simulink model "ALL_SET_GET_SETUP_Funcitons_Library_2020a"  (R2021b)
settings: Solver=VariableStepAuto  StartTime=0.0  StopTime=inf  RelTol=1e-3
(part 1 of 3)
settings Model: Creator=ccortez  LastModifiedBy=SL_1
settings SolverCC: AlgebraicLoopSolver=TrustRegion
settings DebuggingCC: SFMachineParentedDataDiag=warning

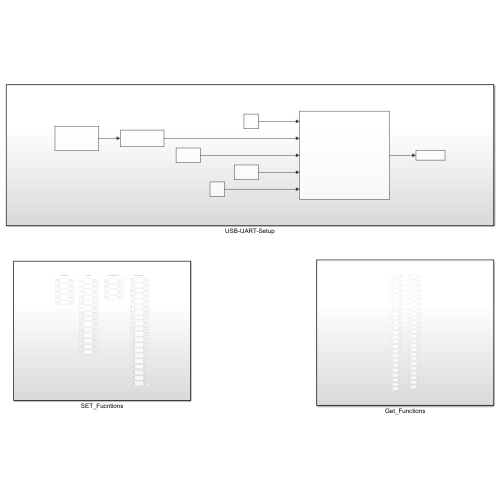
[thumbnail: Simulink's stored preview of the top-level diagram]
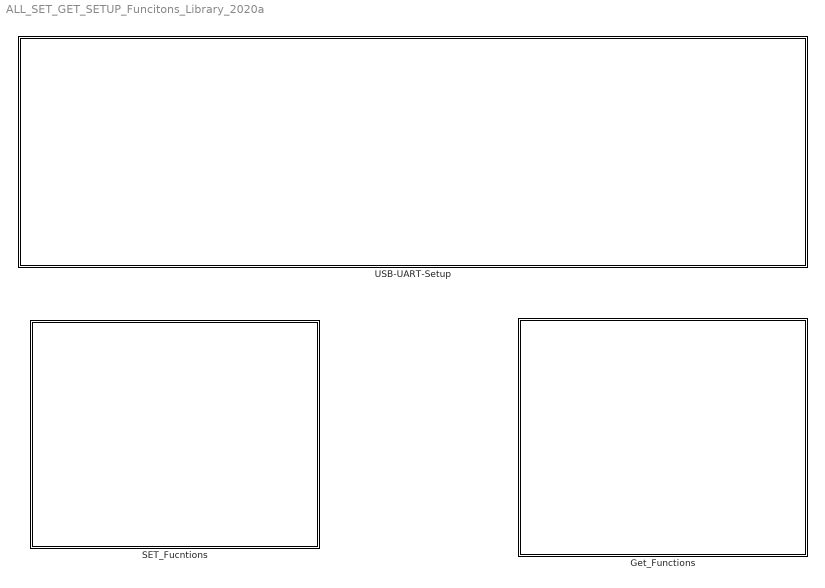
== system ALL_SET_GET_SETUP_Funcitons_Library_2020a ==
  Get_Functions : Subsystem
  SET_Fucntions : Subsystem
  USB-UART-Setup : Subsystem

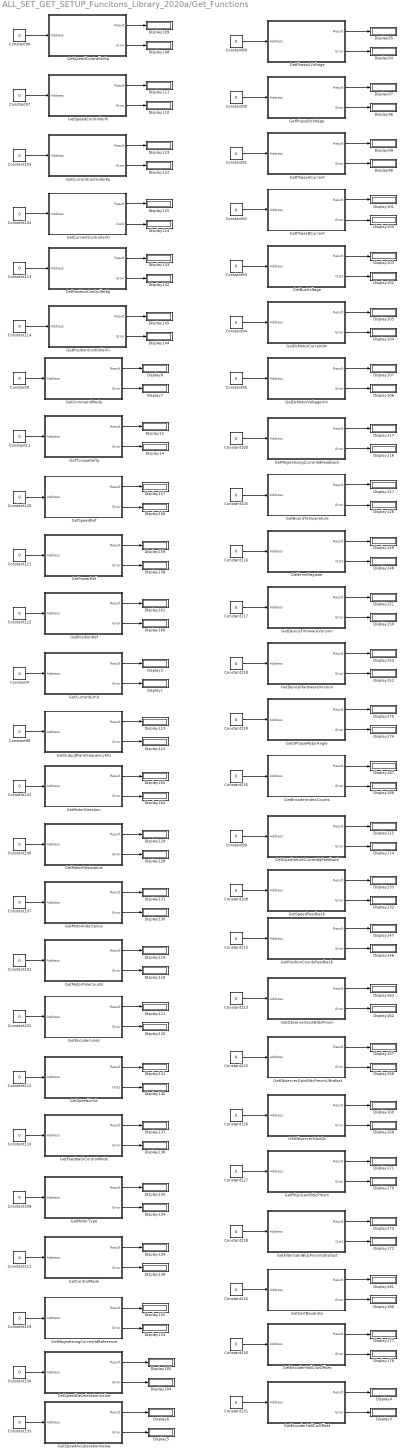
== system ALL_SET_GET_SETUP_Funcitons_Library_2020a/Get_Functions ==
  Constant{4,8,11,89..135} (50 alike) : Constant  Value=0  OutDataTypeStr=uint8
  Display{1..8,14..15,94..177,180..181,184..187} (100 alike) : Display
      settings: Format=decimal (Stored Integer)
  Get3PhaseMotorAngle : Subsystem
  GetBoardTemperature : Subsystem
  GetBusVoltage : Subsystem
  GetCommandMode : Subsystem
  GetControlMode : Subsystem
  GetCurrentControllerKi : Subsystem
  GetCurrentControllerKp : Subsystem
  GetCurrentLimit : Subsystem
  GetDcMotorCurrentIm : Subsystem
  GetDcMotorVoltageVm : Subsystem
  GetDeviceFirmwareVersion : Subsystem
  GetDeviceHardwareVersion : Subsystem
  GetEncoderHallCcwOffset : Subsystem
  GetEncoderHallCwOffset : Subsystem
  GetEncoderIndexCounts : Subsystem
  GetEncoderLines : Subsystem
  GetErrorRegister : Subsystem
  GetFeedbackControlMode : Subsystem
  GetFilterGainBldcPmsm : Subsystem
  GetFilterGainBldcPmsmUltrafast : Subsystem
  GetMagnetizingCurrentIdFeedback : Subsystem
  GetMagnetizingCurrentIdReference : Subsystem
  GetMotorDirection : Subsystem
  GetMotorInductance : Subsystem
  GetMotorPoleCounts : Subsystem
  GetMotorResistance : Subsystem
  GetMotorType : Subsystem
  GetObserverGainBldcPmsm : Subsystem
  GetObserverGainBldcPmsmUltrafast : Subsystem
  GetObserverGainDc : Subsystem
  GetOutputPwmFrequencyKhz : Subsystem
  GetPhaseACurrent : Subsystem
  GetPhaseAVoltage : Subsystem
  GetPhaseBCurrent : Subsystem
  GetPhaseBVoltage : Subsystem
  GetPositionControllerKi : Subsystem
  GetPositionControllerKp : Subsystem
  GetPositionCountsFeedback : Subsystem
  GetPositionRef : Subsystem
  GetPowerRef : Subsystem
  GetQuadratureCurrentIqFeedback : Subsystem
  GetSpeedAccelerationValue : Subsystem
  GetSpeedControllerKi : Subsystem
  GetSpeedControllerKp : Subsystem
  GetSpeedDecelerationValue : Subsystem
  GetSpeedFeedback : Subsystem
  GetSpeedLimit : Subsystem
  GetSpeedRef : Subsystem
  GetTorqueRefIq : Subsystem
  GetUartBaudrate : Subsystem
  wires:
  GetErrorRegister/1(Result) -> Display149/1
  Get3PhaseMotorAngle/2(Error) -> Display174/1
  GetDeviceHardwareVersion/1(Result) -> Display153/1
  Constant91/1 -> GetPhaseACurrent/1(Address)
  GetMagnetizingCurrentIdFeedback/2(Error) -> Display116/1
  Constant129/1 -> Get3PhaseMotorAngle/1(Address)
  GetDcMotorVoltageVm/2(Error) -> Display106/1
  GetPhaseACurrent/1(Result) -> Display99/1
  GetBusVoltage/1(Result) -> Display103/1
  GetErrorRegister/2(Out2) -> Display148/1
  Get3PhaseMotorAngle/1(Result) -> Display175/1
  Constant99/1 -> GetQuadratureCurrentIqFeedback/1(Address)
  Constant117/1 -> GetDeviceFirmwareVersion/1(Address)
  GetPhaseAVoltage/2(Error) -> Display94/1
  Constant116/1 -> GetErrorRegister/1(Address)
  GetPhaseACurrent/2(Error) -> Display98/1
  GetBoardTemperature/1(Result) -> Display127/1
  GetBusVoltage/2(Out2) -> Display102/1
  GetMagnetizingCurrentIdFeedback/1(Result) -> Display117/1
  GetBoardTemperature/2(Error) -> Display126/1
  Constant100/1 -> GetMagnetizingCurrentIdFeedback/1(Address)
  GetPositionCountsFeedback/2(Error) -> Display146/1
  GetPositionCountsFeedback/1(Result) -> Display147/1
  Constant105/1 -> GetBoardTemperature/1(Address)
  GetPhaseBVoltage/1(Result) -> Display97/1
  Constant90/1 -> GetPhaseBVoltage/1(Address)
  GetPhaseBVoltage/2(Error) -> Display96/1
  GetQuadratureCurrentIqFeedback/1(Result) -> Display115/1
  GetDeviceFirmwareVersion/1(Result) -> Display151/1
  GetDcMotorVoltageVm/1(Result) -> Display107/1
  Constant92/1 -> GetPhaseBCurrent/1(Address)
  GetEncoderIndexCounts/1(Result) -> Display187/1
  GetSpeedFeedback/2(Error) -> Display132/1
  GetQuadratureCurrentIqFeedback/2(Error) -> Display114/1
  Constant89/1 -> GetPhaseAVoltage/1(Address)
  GetDeviceFirmwareVersion/2(Error) -> Display150/1
  GetPhaseBCurrent/1(Result) -> Display101/1
  Constant95/1 -> GetDcMotorVoltageVm/1(Address)
  GetPhaseBCurrent/2(Error) -> Display100/1
  GetPhaseAVoltage/1(Result) -> Display95/1
  Constant118/1 -> GetDeviceHardwareVersion/1(Address)
  Constant108/1 -> GetSpeedFeedback/1(Address)
  GetSpeedFeedback/1(Result) -> Display133/1
  GetDcMotorCurrentIm/2(Error) -> Display104/1
  Constant93/1 -> GetBusVoltage/1(Address)
  GetEncoderIndexCounts/2(Error) -> Display186/1
  Constant115/1 -> GetPositionCountsFeedback/1(Address)
  GetDcMotorCurrentIm/1(Result) -> Display105/1
  Constant94/1 -> GetDcMotorCurrentIm/1(Address)
  GetDeviceHardwareVersion/2(Error) -> Display152/1
  Constant135/1 -> GetEncoderIndexCounts/1(Address)
  GetObserverGainBldcPmsmUltrafast/2(Error) -> Display166/1
  GetObserverGainBldcPmsmUltrafast/1(Result) -> Display167/1
  Constant125/1 -> GetObserverGainBldcPmsmUltrafast/1(Address)
  GetPositionControllerKi/1(Result) -> Display145/1
  GetPositionControllerKi/2(Error) -> Display144/1
  GetEncoderHallCcwOffset/1(Result) -> Display177/1
  GetEncoderHallCcwOffset/2(Error) -> Display176/1
  GetUartBaudrate/1(Result) -> Display181/1
  Constant132/1 -> GetUartBaudrate/1(Address)
  Constant126/1 -> GetObserverGainDc/1(Address)
  GetControlMode/1(Result) -> Display139/1
  GetControlMode/2(Error) -> Display138/1
  Constant111/1 -> GetControlMode/1(Address)
  GetFeedbackControlMode/2(Error) -> Display136/1
  GetFeedbackControlMode/1(Result) -> Display137/1
  GetSpeedAccelerationValue/2(Error) -> Display5/1
  GetObserverGainDc/1(Result) -> Display169/1
  GetObserverGainBldcPmsm/2(Error) -> Display162/1
  Constant123/1 -> GetObserverGainBldcPmsm/1(Address)
  GetObserverGainBldcPmsm/1(Result) -> Display163/1
  Constant110/1 -> GetFeedbackControlMode/1(Address)
  GetMotorDirection/2(Error) -> Display164/1
  GetEncoderLines/2(Error) -> Display120/1
  Constant119/1 -> GetMagnetizingCurrentIdReference/1(Address)
  Constant122/1 -> GetPositionRef/1(Address)
  Constant107/1 -> GetMotorInductance/1(Address)
  GetMotorInductance/1(Result) -> Display131/1
  Constant127/1 -> GetFilterGainBldcPmsm/1(Address)
  GetSpeedLimit/2(Out2) -> Display140/1
  Constant112/1 -> GetSpeedLimit/1(Address)
  GetFilterGainBldcPmsmUltrafast/2(Out2) -> Display172/1
  GetMotorInductance/2(Error) -> Display130/1
  GetUartBaudrate/2(Error) -> Display180/1
  Constant133/1 -> GetSpeedAccelerationValue/1(Address)
  Constant128/1 -> GetFilterGainBldcPmsmUltrafast/1(Address)
  GetPositionRef/1(Result) -> Display161/1
  Constant124/1 -> GetMotorDirection/1(Address)
  GetMagnetizingCurrentIdReference/2(Error) -> Display154/1
  Constant130/1 -> GetEncoderHallCcwOffset/1(Address)
  GetFilterGainBldcPmsmUltrafast/1(Result) -> Display173/1
  Constant131/1 -> GetEncoderHallCwOffset/1(Address)
  Constant102/1 -> GetEncoderLines/1(Address)
  GetCurrentControllerKp/2(Error) -> Display122/1
  Constant113/1 -> GetPositionControllerKp/1(Address)
  GetCurrentControllerKp/1(Result) -> Display123/1
  Constant98/1 -> GetOutputPwmFrequencyKhz/1(Address)
  GetSpeedDecelerationValue/2(Error) -> Display184/1
  GetObserverGainDc/2(Error) -> Display168/1
  Constant114/1 -> GetPositionControllerKi/1(Address)
  GetSpeedAccelerationValue/1(Result) -> Display6/1
  GetFilterGainBldcPmsm/2(Error) -> Display170/1
  GetPositionRef/2(Error) -> Display160/1
  Constant134/1 -> GetSpeedDecelerationValue/1(Address)
  GetOutputPwmFrequencyKhz/2(Error) -> Display112/1
  Constant104/1 -> GetCurrentControllerKi/1(Address)
  GetCurrentControllerKi/2(Out2) -> Display124/1
  GetCurrentControllerKi/1(Result) -> Display125/1
  Constant103/1 -> GetCurrentControllerKp/1(Address)
  GetPositionControllerKp/1(Result) -> Display143/1
  GetMotorPoleCounts/2(Error) -> Display118/1
  GetPositionControllerKp/2(Error) -> Display142/1
  GetSpeedDecelerationValue/1(Result) -> Display185/1
  GetFilterGainBldcPmsm/1(Result) -> Display171/1
  GetOutputPwmFrequencyKhz/1(Result) -> Display113/1
  GetEncoderLines/1(Result) -> Display121/1
  GetMotorPoleCounts/1(Result) -> Display119/1
  GetMotorResistance/1(Result) -> Display129/1
  Constant101/1 -> GetMotorPoleCounts/1(Address)
  GetMotorDirection/1(Result) -> Display165/1
  GetMagnetizingCurrentIdReference/1(Result) -> Display155/1
  GetMotorType/1(Result) -> Display135/1
  GetMotorType/2(Error) -> Display134/1
  GetSpeedLimit/1(Result) -> Display141/1
  Constant109/1 -> GetMotorType/1(Address)
  Constant106/1 -> GetMotorResistance/1(Address)
  GetMotorResistance/2(Error) -> Display128/1
  GetPowerRef/2(Error) -> Display158/1
  Constant121/1 -> GetPowerRef/1(Address)
  Constant120/1 -> GetSpeedRef/1(Address)
  GetSpeedRef/1(Result) -> Display157/1
  GetSpeedRef/2(Error) -> Display156/1
  GetTorqueRefIq/1(Result) -> Display15/1
  Constant8/1 -> GetCommandMode/1(Address)
  GetCommandMode/2(Error) -> Display7/1
  GetTorqueRefIq/2(Error) -> Display14/1
  GetPowerRef/1(Result) -> Display159/1
  Constant11/1 -> GetTorqueRefIq/1(Address)
  GetCommandMode/1(Result) -> Display8/1
  Constant4/1 -> GetCurrentLimit/1(Address)
  GetCurrentLimit/1(Result) -> Display2/1
  GetCurrentLimit/2(Error) -> Display1/1
  GetSpeedControllerKi/1(Result) -> Display111/1
  GetSpeedControllerKp/2(Error) -> Display108/1
  GetSpeedControllerKp/1(Result) -> Display109/1
  GetSpeedControllerKi/2(Error) -> Display110/1
  Constant97/1 -> GetSpeedControllerKi/1(Address)
  Constant96/1 -> GetSpeedControllerKp/1(Address)
  GetEncoderHallCwOffset/2(Error) -> Display3/1
  GetEncoderHallCwOffset/1(Result) -> Display4/1

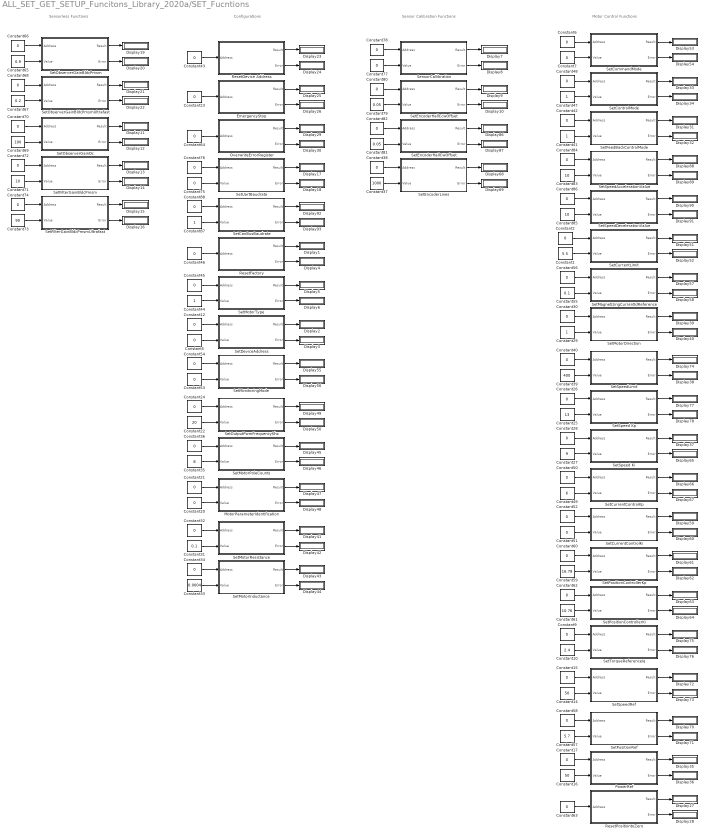
== system ALL_SET_GET_SETUP_Funcitons_Library_2020a/SET_Fucntions ==
  note: Sensor Calibration Functions
  note: Sensorless Functions
  note: Configurations
  note: Motor Control Functions
  Constant1 : Constant  Value=5.5  OutDataTypeStr=single
  Constant10 : Constant  Value=2.4  OutDataTypeStr=single
  Constant{2,5..6,9,12,15,17,21,23..24,26,28,30,32,34,36,38,40,42..43,45..46,48,50,52,54,56,58,60,62..64,66,68,70,72,74,76..78,80,82,84,86,88} (45 alike) : Constant  Value=0  OutDataTypeStr=uint8
  Constant14 : Constant  Value=50  OutDataTypeStr=uint32
  Constant16 : Constant  Value=50  OutDataTypeStr=single
  Constant{7,20,53,75} (4 alike) : Constant  Value=0  OutDataTypeStr=boolean
  Constant22 : Constant  Value=20  OutDataTypeStr=uint32
  Constant25 : Constant  Value=13  OutDataTypeStr=single
  Constant27 : Constant  Value=9  OutDataTypeStr=single
  Constant29 : Constant  OutDataTypeStr=boolean
  Constant31 : Constant  Value=0.1  OutDataTypeStr=single
  Constant33 : Constant  Value=0.0004  OutDataTypeStr=single
  Constant35 : Constant  Value=8  OutDataTypeStr=uint32
  Constant37 : Constant  Value=1000  OutDataTypeStr=uint32
  Constant39 : Constant  Value=400  OutDataTypeStr=uint32
  Constant{41,44,47,87} (4 alike) : Constant  OutDataTypeStr=uint8
  Constant49 : Constant  Value=6  OutDataTypeStr=single
  Constant51 : Constant  Value=0  OutDataTypeStr=single
  Constant55 : Constant  Value=0.1  OutDataTypeStr=single
  Constant57 : Constant  Value=5.7  OutDataTypeStr=uint32
  Constant59 : Constant  Value=16.78  OutDataTypeStr=single
  Constant61 : Constant  Value=10.76  OutDataTypeStr=single
  Constant65 : Constant  Value=0.9  OutDataTypeStr=single
  Constant67 : Constant  Value=0.2  OutDataTypeStr=single
  Constant69 : Constant  Value=100  OutDataTypeStr=single
  Constant71 : Constant  Value=10  OutDataTypeStr=single
  Constant73 : Constant  Value=90  OutDataTypeStr=single
  Constant79 : Constant  Value=0.05  OutDataTypeStr=single
  Constant81 : Constant  Value=0.05  OutDataTypeStr=single
  Constant83 : Constant  Value=10  OutDataTypeStr=single
  Constant85 : Constant  Value=10  OutDataTypeStr=single
  Display{1..78,86..93} (86 alike) : Display
      settings: Format=decimal (Stored Integer)
  EmergencyStop : Subsystem
  MotorParameterIdentification : Subsystem
  OverwriteErrorRegister : Subsystem
  PowerRef : Subsystem
  ResetDevice Address : Subsystem
  ResetFactory : Subsystem
  ResetPositiontoZero : Subsystem
  SensorCallibration : Subsystem
  SetCanBusBaudrate : Subsystem
  SetCommandMode : Subsystem
  SetControlMode : Subsystem
  SetCurrentControlKi : Subsystem
  SetCurrentControlKp : Subsystem
  SetCurrentLimit : Subsystem
  SetDeviceAddress : Subsystem
  SetEncoderHallCcwOffset : Subsystem
  SetEncoderHallCwOffset : Subsystem
  SetEncoderLines : Subsystem
  SetFeedBackControlMode : Subsystem
  SetFilterGainBldcPmsm : Subsystem
  SetFilterGainBldcPmsmUltrafast : Subsystem
  SetMagnetizingCurrentIdReference : Subsystem
  SetMonitoringMode : Subsystem
  SetMotorDirection : Subsystem
  SetMotorInductance : Subsystem
  SetMotorPoleCounts : Subsystem
  SetMotorResistance : Subsystem
  SetMotorType : Subsystem
  SetObserverGainBldcPmsm : Subsystem
  SetObserverGainBldcPmsmUltrafast : Subsystem
  SetObserverGainDc : Subsystem
  SetOutputPwmFrequencyKhz : Subsystem
  SetPositionControllerKi : Subsystem
  SetPositionControllerKp : Subsystem
  SetPositionRef : Subsystem
  SetSpeed Ki : Subsystem
  SetSpeed Kp : Subsystem
  SetSpeedAccelerationValue : Subsystem
  SetSpeedDecelerationValue : Subsystem
  SetSpeedLimit : Subsystem
  SetSpeedRef : Subsystem
  SetTorqueReferenceIq : Subsystem
  SetUartBaudrate : Subsystem
  wires:
  Constant37/1 -> SetEncoderLines/2(Value)
  Constant59/1 -> SetPositionControllerKp/2(Value)
  Constant70/1 -> SetObserverGainDc/1(Address)
  Constant76/1 -> SetUartBaudrate/1(Address)
  Constant35/1 -> SetMotorPoleCounts/2(Value)
  Constant75/1 -> SetUartBaudrate/2(Value)
  Constant68/1 -> SetObserverGainBldcPmsmUltrafast/1(Address)
  Constant61/1 -> SetPositionControllerKi/2(Value)
  Constant72/1 -> SetFilterGainBldcPmsm/1(Address)
  Constant47/1 -> SetControlMode/2(Value)
  Constant54/1 -> SetMonitoringMode/1(Address)
  Constant62/1 -> SetPositionControllerKi/1(Address)
  Constant26/1 -> SetSpeed Kp/1(Address)
  Constant69/1 -> SetObserverGainDc/2(Value)
  Constant71/1 -> SetFilterGainBldcPmsm/2(Value)
  Constant66/1 -> SetObserverGainBldcPmsm/1(Address)
  Constant39/1 -> SetSpeedLimit/2(Value)
  Constant45/1 -> SetMotorType/1(Address)
  Constant40/1 -> SetSpeedLimit/1(Address)
  Constant36/1 -> SetMotorPoleCounts/1(Address)
  Constant17/1 -> PowerRef/1(Address)
  Constant53/1 -> SetMonitoringMode/2(Value)
  Constant16/1 -> PowerRef/2(Value)
  Constant63/1 -> ResetPositiontoZero/1(Address)
  Constant49/1 -> SetCurrentControlKp/2(Value)
  Constant20/1 -> MotorParameterIdentification/2(Value)
  Constant33/1 -> SetMotorInductance/2(Value)
  Constant23/1 -> EmergencyStop/1(Address)
  Constant42/1 -> SetFeedBackControlMode/1(Address)
  Constant25/1 -> SetSpeed Kp/2(Value)
  Constant44/1 -> SetMotorType/2(Value)
  Constant30/1 -> SetMotorDirection/1(Address)
  Constant67/1 -> SetObserverGainBldcPmsmUltrafast/2(Value)
  Constant34/1 -> SetMotorInductance/1(Address)
  Constant24/1 -> SetOutputPwmFrequencyKhz/1(Address)
  Constant21/1 -> MotorParameterIdentification/1(Address)
  Constant28/1 -> SetSpeed Ki/1(Address)
  Constant27/1 -> SetSpeed Ki/2(Value)
  Constant41/1 -> SetFeedBackControlMode/2(Value)
  Constant43/1 -> ResetDevice Address/1(Address)
  Constant38/1 -> SetEncoderLines/1(Address)
  Constant22/1 -> SetOutputPwmFrequencyKhz/2(Value)
  Constant29/1 -> SetMotorDirection/2(Value)
  Constant55/1 -> SetMagnetizingCurrentIdReference/2(Value)
  Constant56/1 -> SetMagnetizingCurrentIdReference/1(Address)
  Constant52/1 -> SetCurrentControlKi/1(Address)
  Constant51/1 -> SetCurrentControlKi/2(Value)
  Constant73/1 -> SetFilterGainBldcPmsmUltrafast/2(Value)
  Constant74/1 -> SetFilterGainBldcPmsmUltrafast/1(Address)
  Constant60/1 -> SetPositionControllerKp/1(Address)
  Constant48/1 -> SetControlMode/1(Address)
  Constant15/1 -> SetSpeedRef/1(Address)
  Constant14/1 -> SetSpeedRef/2(Value)
  Constant32/1 -> SetMotorResistance/1(Address)
  Constant31/1 -> SetMotorResistance/2(Value)
  Constant50/1 -> SetCurrentControlKp/1(Address)
  Constant46/1 -> ResetFactory/1(Address)
  Constant77/1 -> SensorCallibration/2(Value)
  Constant65/1 -> SetObserverGainBldcPmsm/2(Value)
  Constant78/1 -> SensorCallibration/1(Address)
  Constant64/1 -> OverwriteErrorRegister/1(Address)
  Constant57/1 -> SetPositionRef/2(Value)
  Constant58/1 -> SetPositionRef/1(Address)
  Constant79/1 -> SetEncoderHallCcwOffset/2(Value)
  Constant80/1 -> SetEncoderHallCcwOffset/1(Address)
  Constant6/1 -> SetCommandMode/1(Address)
  Constant9/1 -> SetTorqueReferenceIq/1(Address)
  Constant10/1 -> SetTorqueReferenceIq/2(Value)
  Constant7/1 -> SetCommandMode/2(Value)
  SetDeviceAddress/2(Error) -> Display3/1
  Constant5/1 -> SetDeviceAddress/2(Value)
  Constant12/1 -> SetDeviceAddress/1(Address)
  Constant1/1 -> SetCurrentLimit/2(Value)
  SetDeviceAddress/1(Result) -> Display2/1
  Constant2/1 -> SetCurrentLimit/1(Address)
  Constant82/1 -> SetEncoderHallCwOffset/1(Address)
  Constant81/1 -> SetEncoderHallCwOffset/2(Value)
  SetCanBusBaudrate/2(Error) -> Display93/1
  SetCanBusBaudrate/1(Result) -> Display92/1
  SetEncoderHallCwOffset/1(Result) -> Display86/1
  SetEncoderHallCwOffset/2(Error) -> Display87/1
  Constant87/1 -> SetCanBusBaudrate/2(Value)
  Constant85/1 -> SetSpeedDecelerationValue/2(Value)
  Constant88/1 -> SetCanBusBaudrate/1(Address)
  SetSpeedAccelerationValue/2(Error) -> Display89/1
  Constant84/1 -> SetSpeedAccelerationValue/1(Address)
  SetSpeedAccelerationValue/1(Result) -> Display88/1
  SetSpeedDecelerationValue/2(Error) -> Display91/1
  Constant83/1 -> SetSpeedAccelerationValue/2(Value)
  Constant86/1 -> SetSpeedDecelerationValue/1(Address)
  SetSpeedDecelerationValue/1(Result) -> Display90/1
  ResetFactory/2(Error) -> Display4/1
  ResetFactory/1(Result) -> Display1/1
  SetMotorType/2(Error) -> Display6/1
  SetMotorType/1(Result) -> Display5/1
  SensorCallibration/1(Result) -> Display7/1
  SetEncoderHallCcwOffset/1(Result) -> Display9/1
  SensorCallibration/2(Error) -> Display8/1
  SetEncoderHallCcwOffset/2(Error) -> Display10/1
  SetFilterGainBldcPmsm/2(Error) -> Display14/1
  SetFilterGainBldcPmsmUltrafast/1(Result) -> Display15/1
  SetObserverGainDc/2(Error) -> Display12/1
  SetFilterGainBldcPmsm/1(Result) -> Display13/1
  SetUartBaudrate/2(Error) -> Display18/1
  SetUartBaudrate/1(Result) -> Display17/1
  SetObserverGainDc/1(Result) -> Display11/1
  SetFilterGainBldcPmsmUltrafast/2(Error) -> Display16/1
  SetObserverGainBldcPmsm/1(Result) -> Display19/1
  SetObserverGainBldcPmsmUltrafast/1(Result) -> Display21/1
  SetObserverGainBldcPmsm/2(Error) -> Display20/1
  SetObserverGainBldcPmsmUltrafast/2(Error) -> Display22/1
  EmergencyStop/2(Error) -> Display26/1
  ResetPositiontoZero/1(Result) -> Display27/1
  ResetDevice Address/2(Error) -> Display24/1
  EmergencyStop/1(Result) -> Display25/1
  OverwriteErrorRegister/2(Error) -> Display30/1
  OverwriteErrorRegister/1(Result) -> Display29/1
  ResetDevice Address/1(Result) -> Display23/1
  ResetPositiontoZero/2(Error) -> Display28/1
  SetFeedBackControlMode/1(Result) -> Display31/1
  SetFeedBackControlMode/2(Error) -> Display32/1
  SetControlMode/1(Result) -> Display33/1
  SetControlMode/2(Error) -> Display34/1
  PowerRef/2(Error) -> Display36/1
  PowerRef/1(Result) -> Display35/1
  SetPositionControllerKi/1(Result) -> Display63/1
  SetCurrentControlKi/2(Error) -> Display60/1
  SetCurrentControlKi/1(Result) -> Display59/1
  SetSpeed Ki/1(Result) -> Display37/1
  SetCurrentControlKp/1(Result) -> Display66/1
  SetSpeed Ki/2(Error) -> Display65/1
  SetCurrentControlKp/2(Error) -> Display67/1
  SetOutputPwmFrequencyKhz/2(Error) -> Display50/1
  MotorParameterIdentification/2(Error) -> Display48/1
  SetCurrentLimit/2(Error) -> Display52/1
  SetCommandMode/2(Error) -> Display54/1
  SetCurrentLimit/1(Result) -> Display51/1
  SetPositionControllerKp/1(Result) -> Display61/1
  SetCommandMode/1(Result) -> Display53/1
  SetSpeedRef/2(Error) -> Display73/1
  SetPositionControllerKp/2(Error) -> Display62/1
  SetMagnetizingCurrentIdReference/1(Result) -> Display57/1
  SetPositionRef/2(Error) -> Display71/1
  SetTorqueReferenceIq/1(Result) -> Display75/1
  SetTorqueReferenceIq/2(Error) -> Display76/1
  SetSpeedRef/1(Result) -> Display72/1
  SetSpeed Kp/2(Error) -> Display78/1
  SetSpeed Kp/1(Result) -> Display77/1
  SetMagnetizingCurrentIdReference/2(Error) -> Display58/1
  SetPositionRef/1(Result) -> Display70/1
  SetOutputPwmFrequencyKhz/1(Result) -> Display49/1
  SetMotorInductance/1(Result) -> Display43/1
  SetMotorInductance/2(Error) -> Display44/1
  SetMotorPoleCounts/2(Error) -> Display46/1
  SetMonitoringMode/2(Error) -> Display56/1
  SetMotorPoleCounts/1(Result) -> Display45/1
  SetPositionControllerKi/2(Error) -> Display64/1
  SetMotorDirection/1(Result) -> Display39/1
  SetMonitoringMode/1(Result) -> Display55/1
  SetMotorResistance/2(Error) -> Display42/1
  SetMotorResistance/1(Result) -> Display41/1
  SetEncoderLines/1(Result) -> Display68/1
  SetSpeedLimit/2(Error) -> Display38/1
  SetSpeedLimit/1(Result) -> Display74/1
  MotorParameterIdentification/1(Result) -> Display47/1
  SetEncoderLines/2(Error) -> Display69/1
  SetMotorDirection/2(Error) -> Display40/1

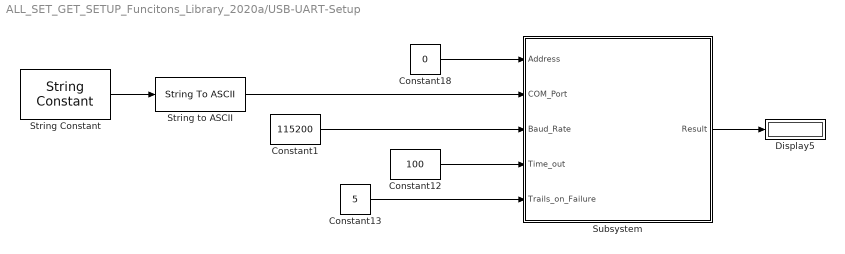
== system ALL_SET_GET_SETUP_Funcitons_Library_2020a/USB-UART-Setup ==
  Constant1 : Constant  Value=115200  OutDataTypeStr=uint32
  Constant12 : Constant  Value=100  OutDataTypeStr=double
  Constant13 : Constant  Value=5  OutDataTypeStr=int32
  Constant18 : Constant  Value=0  OutDataTypeStr=uint8
  Display5 : Display
      settings: Format=decimal (Stored Integer)
  String Constant : StringConstant  String="\"COM6\""
  String to ASCII : StringToASCII  OutputVectorSize=5
  Subsystem : Subsystem
  wires:
  String Constant/1 -> String to ASCII/1
  Constant18/1 -> Subsystem/1(Address)
  String to ASCII/1 -> Subsystem/2(COM_Port)
  Constant1/1 -> Subsystem/3(Baud_Rate)
  Constant12/1 -> Subsystem/4(Time_out)
  Constant13/1 -> Subsystem/5(Trails_on_Failure)
  Subsystem/1(Result) -> Display5/1

== system ALL_SET_GET_SETUP_Funcitons_Library_2020a/Get_Functions/Get3PhaseMotorAngle ==
  Address : Inport
  S-Function Builder87 : S-Function  Priority=3  FunctionName=Get3PhaseMotorAngle  SFunctionModules=Get3PhaseMotorAngle_wrapper  SFunctionDeploymentMode=off  EnableBusSupport=off  mask(S-Function Builder){}
      mask help: Simulink:masks:SFunctionBuilder_MD
      mask init:
      | val = [[.9  0.75 0.75 1 1 .9 .9 1]',[1 1 0.75 0.75 .9 .9 1 .9]'];try , sys = get_param(gcb,'SfunBuilderFcnName');if isempty(sys), sys = get_param(gcb,'FunctionName'); end,catch, sys = get_param(gcb,'FunctionName'); end
      settings: CopyFcn=set_param(gcbh,'LinkStatus','none')  OpenFcn=sfunctionwizard(gcbh)
      mask Display: plot(val(:,1),val(:,2)),disp(sys),port_label('input',1,'Address'),port_label('output',1,'Result'),port_label('output',2,'Error')
  Result : Outport
  Error : Outport  Port=2
  wires:
  Address/1 -> S-Function Builder87/1
  S-Function Builder87/1 -> Result/1
  S-Function Builder87/2 -> Error/1

== system ALL_SET_GET_SETUP_Funcitons_Library_2020a/Get_Functions/GetBoardTemperature ==
  Address : Inport
  S-Function Builder63 : S-Function  Priority=3  FunctionName=GetBoardTemperature  SFunctionModules=GetBoardTemperature_wrapper  SFunctionDeploymentMode=off  EnableBusSupport=off  mask(S-Function Builder){}
      mask help: Simulink:masks:SFunctionBuilder_MD
      mask init: same as ALL_SET_GET_SETUP_Funcitons_Library_2020a/Get_Functions/Get3PhaseMotorAngle/S-Function Builder87
      settings: CopyFcn=set_param(gcbh,'LinkStatus','none')  OpenFcn=sfunctionwizard(gcbh)
      mask Display: plot(val(:,1),val(:,2)),disp(sys),port_label('input',1,'Address'),port_label('output',1,'Result'),port_label('output',2,'Error')
  Result : Outport
  Error : Outport  Port=2
  wires:
  Address/1 -> S-Function Builder63/1
  S-Function Builder63/1 -> Result/1
  S-Function Builder63/2 -> Error/1

== system ALL_SET_GET_SETUP_Funcitons_Library_2020a/Get_Functions/GetBusVoltage ==
  Address : Inport
  S-Function Builder51 : S-Function  Priority=3  FunctionName=GetBusVoltage  SFunctionModules=GetBusVoltage_wrapper  SFunctionDeploymentMode=off  EnableBusSupport=off  mask(S-Function Builder){}
      mask help: Simulink:masks:SFunctionBuilder_MD
      mask init: same as ALL_SET_GET_SETUP_Funcitons_Library_2020a/Get_Functions/Get3PhaseMotorAngle/S-Function Builder87
      settings: CopyFcn=set_param(gcbh,'LinkStatus','none')  OpenFcn=sfunctionwizard(gcbh)
      mask Display:
      | plot(val(:,1),val(:,2))
      | disp(sys)
      | port_label('input',1,'Address')
      | port_label('output',1,'Result')
      | port_label('output',2,'Error')
  Result : Outport
  Out2 : Outport  Port=2
  wires:
  S-Function Builder51/2 -> Out2/1
  Address/1 -> S-Function Builder51/1
  S-Function Builder51/1 -> Result/1

== system ALL_SET_GET_SETUP_Funcitons_Library_2020a/Get_Functions/GetCommandMode ==
  Address : Inport
  S-Function Builder3 : S-Function  Priority=3  FunctionName=GetCommandMode  SFunctionModules=GetCommandMode_wrapper  SFunctionDeploymentMode=off  EnableBusSupport=off  mask(S-Function Builder){}
      mask help: Simulink:masks:SFunctionBuilder_MD
      mask init: same as ALL_SET_GET_SETUP_Funcitons_Library_2020a/Get_Functions/Get3PhaseMotorAngle/S-Function Builder87
      settings: CopyFcn=set_param(gcbh,'LinkStatus','none')  OpenFcn=sfunctionwizard(gcbh)
      mask Display:
      | plot(val(:,1),val(:,2))
      | disp(sys)
      | port_label('input',1,'Address')
      | port_label('output',1,'Result')
      | port_label('output',2,'Error')
  Result : Outport
  Error : Outport  Port=2
  wires:
  S-Function Builder3/2 -> Error/1
  S-Function Builder3/1 -> Result/1
  Address/1 -> S-Function Builder3/1

== system ALL_SET_GET_SETUP_Funcitons_Library_2020a/Get_Functions/GetControlMode ==
  Address : Inport
  S-Function Builder69 : S-Function  Priority=3  FunctionName=GetControlMode  SFunctionModules=GetControlMode_wrapper  SFunctionDeploymentMode=off  EnableBusSupport=off  mask(S-Function Builder){}
      mask help: Simulink:masks:SFunctionBuilder_MD
      mask init: same as ALL_SET_GET_SETUP_Funcitons_Library_2020a/Get_Functions/Get3PhaseMotorAngle/S-Function Builder87
      settings: CopyFcn=set_param(gcbh,'LinkStatus','none')  OpenFcn=sfunctionwizard(gcbh)
      mask Display: plot(val(:,1),val(:,2)),disp(sys),port_label('input',1,'Address'),port_label('output',1,'Result'),port_label('output',2,'Error')
  Result : Outport
  Error : Outport  Port=2
  wires:
  Address/1 -> S-Function Builder69/1
  S-Function Builder69/1 -> Result/1
  S-Function Builder69/2 -> Error/1

== system ALL_SET_GET_SETUP_Funcitons_Library_2020a/Get_Functions/GetCurrentControllerKi ==
  Address : Inport
  S-Function Builder62 : S-Function  Priority=3  FunctionName=GetCurrentControllerKi  SFunctionModules=GetCurrentControllerKi_wrapper  SFunctionDeploymentMode=off  EnableBusSupport=off  mask(S-Function Builder){}
      mask help: Simulink:masks:SFunctionBuilder_MD
      mask init: same as ALL_SET_GET_SETUP_Funcitons_Library_2020a/Get_Functions/Get3PhaseMotorAngle/S-Function Builder87
      settings: CopyFcn=set_param(gcbh,'LinkStatus','none')  OpenFcn=sfunctionwizard(gcbh)
      mask Display: plot(val(:,1),val(:,2)),disp(sys),port_label('input',1,'Address'),port_label('output',1,'Result'),port_label('output',2,'Error')
  Result : Outport
  Out2 : Outport  Port=2
  wires:
  S-Function Builder62/2 -> Out2/1
  S-Function Builder62/1 -> Result/1
  Address/1 -> S-Function Builder62/1

== system ALL_SET_GET_SETUP_Funcitons_Library_2020a/Get_Functions/GetCurrentControllerKp ==
  Address : Inport
  S-Function Builder61 : S-Function  Priority=3  FunctionName=GetCurrentControllerKp  SFunctionModules=GetCurrentControllerKp_wrapper  SFunctionDeploymentMode=off  EnableBusSupport=off  mask(S-Function Builder){}
      mask help: Simulink:masks:SFunctionBuilder_MD
      mask init: same as ALL_SET_GET_SETUP_Funcitons_Library_2020a/Get_Functions/Get3PhaseMotorAngle/S-Function Builder87
      settings: CopyFcn=set_param(gcbh,'LinkStatus','none')  OpenFcn=sfunctionwizard(gcbh)
      mask Display:
      | plot(val(:,1),val(:,2))
      | disp(sys)
      | port_label('input',1,'Address')
      | port_label('output',1,'Result')
      | port_label('output',2,'Error')
  Result : Outport
  Error : Outport  Port=2
  wires:
  S-Function Builder61/2 -> Error/1
  S-Function Builder61/1 -> Result/1
  Address/1 -> S-Function Builder61/1

== system ALL_SET_GET_SETUP_Funcitons_Library_2020a/Get_Functions/GetCurrentLimit ==
  Address : Inport
  Display11 : Display
      settings: Format=decimal (Stored Integer)
  Display9 : Display
      settings: Format=decimal (Stored Integer)
  S-Function Builder6 : S-Function  Priority=3  FunctionName=GetCurrentLimit  SFunctionModules=GetCurrentLimit_wrapper  SFunctionDeploymentMode=off  EnableBusSupport=off  mask(S-Function Builder){}
      mask help: Simulink:masks:SFunctionBuilder_MD
      mask init: same as ALL_SET_GET_SETUP_Funcitons_Library_2020a/Get_Functions/Get3PhaseMotorAngle/S-Function Builder87
      settings: CopyFcn=set_param(gcbh,'LinkStatus','none')  OpenFcn=sfunctionwizard(gcbh)
      mask Display: plot(val(:,1),val(:,2)),disp(sys),port_label('input',1,'Address'),port_label('output',1,'Result'),port_label('output',2,'Error')
  Result : Outport  OutDataTypeStr=single  LockScale=on
  Error : Outport  Port=2  OutDataTypeStr=int32  LockScale=on
  wires:
  S-Function Builder6/1 -> Result/1, Display9/1
  Address/1 -> S-Function Builder6/1
  S-Function Builder6/2 -> Error/1, Display11/1

== system ALL_SET_GET_SETUP_Funcitons_Library_2020a/Get_Functions/GetDcMotorCurrentIm ==
  Address : Inport
  S-Function Builder52 : S-Function  Priority=3  FunctionName=GetDcMotorCurrentIm  SFunctionModules=GetDcMotorCurrentIm_wrapper  SFunctionDeploymentMode=off  EnableBusSupport=off  mask(S-Function Builder){}
      mask help: Simulink:masks:SFunctionBuilder_MD
      mask init: same as ALL_SET_GET_SETUP_Funcitons_Library_2020a/Get_Functions/Get3PhaseMotorAngle/S-Function Builder87
      settings: CopyFcn=set_param(gcbh,'LinkStatus','none')  OpenFcn=sfunctionwizard(gcbh)
      mask Display: plot(val(:,1),val(:,2)),disp(sys),port_label('input',1,'Address'),port_label('output',1,'Result'),port_label('output',2,'Error')
  Result : Outport
  Error : Outport  Port=2
  wires:
  S-Function Builder52/1 -> Result/1
  Address/1 -> S-Function Builder52/1
  S-Function Builder52/2 -> Error/1

== system ALL_SET_GET_SETUP_Funcitons_Library_2020a/Get_Functions/GetDcMotorVoltageVm ==
  Address : Inport
  S-Function Builder53 : S-Function  Priority=3  FunctionName=GetDcMotorVoltageVm  SFunctionModules=GetDcMotorVoltageVm_wrapper  SFunctionDeploymentMode=off  EnableBusSupport=off  mask(S-Function Builder){}
      mask help: Simulink:masks:SFunctionBuilder_MD
      mask init: same as ALL_SET_GET_SETUP_Funcitons_Library_2020a/Get_Functions/Get3PhaseMotorAngle/S-Function Builder87
      settings: CopyFcn=set_param(gcbh,'LinkStatus','none')  OpenFcn=sfunctionwizard(gcbh)
      mask Display: plot(val(:,1),val(:,2)),disp(sys),port_label('input',1,'Address'),port_label('output',1,'Result'),port_label('output',2,'Error')
  Result : Outport
  Error : Outport  Port=2
  wires:
  S-Function Builder53/1 -> Result/1
  Address/1 -> S-Function Builder53/1
  S-Function Builder53/2 -> Error/1

== system ALL_SET_GET_SETUP_Funcitons_Library_2020a/Get_Functions/GetDeviceFirmwareVersion ==
  Address : Inport
  S-Function Builder75 : S-Function  Priority=3  FunctionName=GetDeviceFirmwareVersion  SFunctionModules=GetDeviceFirmwareVersion_wrapper  SFunctionDeploymentMode=off  EnableBusSupport=off  mask(S-Function Builder){}
      mask help: Simulink:masks:SFunctionBuilder_MD
      mask init: same as ALL_SET_GET_SETUP_Funcitons_Library_2020a/Get_Functions/Get3PhaseMotorAngle/S-Function Builder87
      settings: CopyFcn=set_param(gcbh,'LinkStatus','none')  OpenFcn=sfunctionwizard(gcbh)
      mask Display: plot(val(:,1),val(:,2)),disp(sys),port_label('input',1,'Address'),port_label('output',1,'Result'),port_label('output',2,'Error')
  Result : Outport
  Error : Outport  Port=2
  wires:
  Address/1 -> S-Function Builder75/1
  S-Function Builder75/1 -> Result/1
  S-Function Builder75/2 -> Error/1

== system ALL_SET_GET_SETUP_Funcitons_Library_2020a/Get_Functions/GetDeviceHardwareVersion ==
  Address : Inport
  S-Function Builder76 : S-Function  Priority=3  FunctionName=GetDeviceHardwareVersion  SFunctionModules=GetDeviceHardwareVersion_wrapper  SFunctionDeploymentMode=off  EnableBusSupport=off  mask(S-Function Builder){}
      mask help: Simulink:masks:SFunctionBuilder_MD
      mask init: same as ALL_SET_GET_SETUP_Funcitons_Library_2020a/Get_Functions/Get3PhaseMotorAngle/S-Function Builder87
      settings: CopyFcn=set_param(gcbh,'LinkStatus','none')  OpenFcn=sfunctionwizard(gcbh)
      mask Display: plot(val(:,1),val(:,2)),disp(sys),port_label('input',1,'Address'),port_label('output',1,'Result'),port_label('output',2,'Error')
  Result : Outport
  Error : Outport  Port=2
  wires:
  S-Function Builder76/2 -> Error/1
  Address/1 -> S-Function Builder76/1
  S-Function Builder76/1 -> Result/1

== system ALL_SET_GET_SETUP_Funcitons_Library_2020a/Get_Functions/GetEncoderHallCcwOffset ==
  Address : Inport
  S-Function Builder88 : S-Function  Priority=3  FunctionName=GetEncoderHallCcwOffset  SFunctionModules=GetEncoderHallCcwOffset_wrapper  SFunctionDeploymentMode=off  EnableBusSupport=off  mask(S-Function Builder){}
      mask help: Simulink:masks:SFunctionBuilder_MD
      mask init: same as ALL_SET_GET_SETUP_Funcitons_Library_2020a/Get_Functions/Get3PhaseMotorAngle/S-Function Builder87
      settings: CopyFcn=set_param(gcbh,'LinkStatus','none')  OpenFcn=sfunctionwizard(gcbh)
      mask Display: plot(val(:,1),val(:,2)),disp(sys),port_label('input',1,'Address'),port_label('output',1,'Result'),port_label('output',2,'Error')
  Result : Outport
  Error : Outport  Port=2
  wires:
  S-Function Builder88/1 -> Result/1
  S-Function Builder88/2 -> Error/1
  Address/1 -> S-Function Builder88/1

== system ALL_SET_GET_SETUP_Funcitons_Library_2020a/Get_Functions/GetEncoderHallCwOffset ==
  Address : Inport
  S-Function Builder89 : S-Function  Priority=3  FunctionName=GetEncoderHallCwOffset  SFunctionModules=GetEncoderHallCwOffset_wrapper  SFunctionDeploymentMode=off  EnableBusSupport=off  mask(S-Function Builder){}
      mask help: Simulink:masks:SFunctionBuilder_MD
      mask init: same as ALL_SET_GET_SETUP_Funcitons_Library_2020a/Get_Functions/Get3PhaseMotorAngle/S-Function Builder87
      settings: CopyFcn=set_param(gcbh,'LinkStatus','none')  OpenFcn=sfunctionwizard(gcbh)
      mask Display: plot(val(:,1),val(:,2)),disp(sys),port_label('input',1,'Address'),port_label('output',1,'Result'),port_label('output',2,'Error')
  Result : Outport
  Error : Outport  Port=2
  wires:
  Address/1 -> S-Function Builder89/1
  S-Function Builder89/1 -> Result/1
  S-Function Builder89/2 -> Error/1

== system ALL_SET_GET_SETUP_Funcitons_Library_2020a/Get_Functions/GetEncoderIndexCounts ==
  Address : Inport
  S-Function Builder93 : S-Function  Priority=3  FunctionName=GetEncoderIndexCounts  SFunctionModules=GetEncoderIndexCounts_wrapper  SFunctionDeploymentMode=off  EnableBusSupport=off  mask(S-Function Builder){}
      mask help: Simulink:masks:SFunctionBuilder_MD
      mask init: same as ALL_SET_GET_SETUP_Funcitons_Library_2020a/Get_Functions/Get3PhaseMotorAngle/S-Function Builder87
      settings: CopyFcn=set_param(gcbh,'LinkStatus','none')  OpenFcn=sfunctionwizard(gcbh)
      mask Display: plot(val(:,1),val(:,2)),disp(sys),port_label('input',1,'Address'),port_label('output',1,'Result'),port_label('output',2,'Error')
  Result : Outport
  Error : Outport  Port=2
  wires:
  S-Function Builder93/1 -> Result/1
  Address/1 -> S-Function Builder93/1
  S-Function Builder93/2 -> Error/1

== system ALL_SET_GET_SETUP_Funcitons_Library_2020a/Get_Functions/GetEncoderLines ==
  Address : Inport
  S-Function Builder60 : S-Function  Priority=3  FunctionName=GetIncrementalEncoderLines  SFunctionModules=GetIncrementalEncoderLines_wrapper  SFunctionDeploymentMode=off  EnableBusSupport=off  mask(S-Function Builder){}
      mask help: Simulink:masks:SFunctionBuilder_MD
      mask init: same as ALL_SET_GET_SETUP_Funcitons_Library_2020a/Get_Functions/Get3PhaseMotorAngle/S-Function Builder87
      settings: CopyFcn=set_param(gcbh,'LinkStatus','none')  OpenFcn=sfunctionwizard(gcbh)
      mask Display:
      | plot(val(:,1),val(:,2))
      | disp(sys)
      | port_label('input',1,'Address')
      | port_label('output',1,'Result')
      | port_label('output',2,'Error')
  Result : Outport
  Error : Outport  Port=2
  wires:
  S-Function Builder60/2 -> Error/1
  S-Function Builder60/1 -> Result/1
  Address/1 -> S-Function Builder60/1

== system ALL_SET_GET_SETUP_Funcitons_Library_2020a/Get_Functions/GetErrorRegister ==
  Address : Inport
  S-Function Builder74 : S-Function  Priority=3  FunctionName=GetErrorRegister  SFunctionModules=GetErrorRegister_wrapper  SFunctionDeploymentMode=off  EnableBusSupport=off  mask(S-Function Builder){}
      mask help: Simulink:masks:SFunctionBuilder_MD
      mask init: same as ALL_SET_GET_SETUP_Funcitons_Library_2020a/Get_Functions/Get3PhaseMotorAngle/S-Function Builder87
      settings: CopyFcn=set_param(gcbh,'LinkStatus','none')  OpenFcn=sfunctionwizard(gcbh)
      mask Display: plot(val(:,1),val(:,2)),disp(sys),port_label('input',1,'Address'),port_label('output',1,'Result'),port_label('output',2,'Error')
  Result : Outport
  Out2 : Outport  Port=2
  wires:
  S-Function Builder74/1 -> Result/1
  Address/1 -> S-Function Builder74/1
  S-Function Builder74/2 -> Out2/1

== system ALL_SET_GET_SETUP_Funcitons_Library_2020a/Get_Functions/GetFeedbackControlMode ==
  Address : Inport
  S-Function Builder68 : S-Function  Priority=3  FunctionName=GetFeedbackControlMode  SFunctionModules=GetFeedbackControlMode_wrapper  SFunctionDeploymentMode=off  EnableBusSupport=off  mask(S-Function Builder){}
      mask help: Simulink:masks:SFunctionBuilder_MD
      mask init: same as ALL_SET_GET_SETUP_Funcitons_Library_2020a/Get_Functions/Get3PhaseMotorAngle/S-Function Builder87
      settings: CopyFcn=set_param(gcbh,'LinkStatus','none')  OpenFcn=sfunctionwizard(gcbh)
      mask Display:
      | plot(val(:,1),val(:,2))
      | disp(sys)
      | port_label('input',1,'Address')
      | port_label('output',1,'Result')
      | port_label('output',2,'Error')
  Result : Outport
  Error : Outport  Port=2
  wires:
  S-Function Builder68/2 -> Error/1
  S-Function Builder68/1 -> Result/1
  Address/1 -> S-Function Builder68/1

== system ALL_SET_GET_SETUP_Funcitons_Library_2020a/Get_Functions/GetFilterGainBldcPmsm ==
  Address : Inport
  S-Function Builder85 : S-Function  Priority=3  FunctionName=GetFilterGainBldcPmsm  SFunctionModules=GetFilterGainBldcPmsm_wrapper  SFunctionDeploymentMode=off  EnableBusSupport=off  mask(S-Function Builder){}
      mask help: Simulink:masks:SFunctionBuilder_MD
      mask init: same as ALL_SET_GET_SETUP_Funcitons_Library_2020a/Get_Functions/Get3PhaseMotorAngle/S-Function Builder87
      settings: CopyFcn=set_param(gcbh,'LinkStatus','none')  OpenFcn=sfunctionwizard(gcbh)
      mask Display: plot(val(:,1),val(:,2)),disp(sys),port_label('input',1,'Address'),port_label('output',1,'Result'),port_label('output',2,'Error')
  Result : Outport
  Error : Outport  Port=2
  wires:
  S-Function Builder85/1 -> Result/1
  Address/1 -> S-Function Builder85/1
  S-Function Builder85/2 -> Error/1

== system ALL_SET_GET_SETUP_Funcitons_Library_2020a/Get_Functions/GetFilterGainBldcPmsmUltrafast ==
  Address : Inport
  S-Function Builder86 : S-Function  Priority=3  FunctionName=GetFilterGainBldcPmsmUltrafast  SFunctionModules=GetFilterGainBldcPmsmUltrafast_wrapper  SFunctionDeploymentMode=off  EnableBusSupport=off  mask(S-Function Builder){}
      mask help: Simulink:masks:SFunctionBuilder_MD
      mask init: same as ALL_SET_GET_SETUP_Funcitons_Library_2020a/Get_Functions/Get3PhaseMotorAngle/S-Function Builder87
      settings: CopyFcn=set_param(gcbh,'LinkStatus','none')  OpenFcn=sfunctionwizard(gcbh)
      mask Display: plot(val(:,1),val(:,2)),disp(sys),port_label('input',1,'Address'),port_label('output',1,'Result'),port_label('output',2,'Error')
  Result : Outport
  Out2 : Outport  Port=2
  wires:
  S-Function Builder86/2 -> Out2/1
  Address/1 -> S-Function Builder86/1
  S-Function Builder86/1 -> Result/1

== system ALL_SET_GET_SETUP_Funcitons_Library_2020a/Get_Functions/GetMagnetizingCurrentIdFeedback ==
  Address : Inport
  S-Function Builder58 : S-Function  Priority=3  FunctionName=GetMagnetizingCurrentIdFeedback  SFunctionModules=GetMagnetizingCurrentIdFeedback_wrapper  SFunctionDeploymentMode=off  EnableBusSupport=off  mask(S-Function Builder){}
      mask help: Simulink:masks:SFunctionBuilder_MD
      mask init: same as ALL_SET_GET_SETUP_Funcitons_Library_2020a/Get_Functions/Get3PhaseMotorAngle/S-Function Builder87
      settings: CopyFcn=set_param(gcbh,'LinkStatus','none')  OpenFcn=sfunctionwizard(gcbh)
      mask Display: plot(val(:,1),val(:,2)),disp(sys),port_label('input',1,'Address'),port_label('output',1,'Result'),port_label('output',2,'Error')
  Result : Outport
  Error : Outport  Port=2
  wires:
  S-Function Builder58/1 -> Result/1
  S-Function Builder58/2 -> Error/1
  Address/1 -> S-Function Builder58/1

== system ALL_SET_GET_SETUP_Funcitons_Library_2020a/Get_Functions/GetMagnetizingCurrentIdReference ==
  Address : Inport
  S-Function Builder77 : S-Function  Priority=3  FunctionName=GetMagnetizingCurrentIdReference  SFunctionModules=GetMagnetizingCurrentIdReference_wrapper  SFunctionDeploymentMode=off  EnableBusSupport=off  mask(S-Function Builder){}
      mask help: Simulink:masks:SFunctionBuilder_MD
      mask init: same as ALL_SET_GET_SETUP_Funcitons_Library_2020a/Get_Functions/Get3PhaseMotorAngle/S-Function Builder87
      settings: CopyFcn=set_param(gcbh,'LinkStatus','none')  OpenFcn=sfunctionwizard(gcbh)
      mask Display: plot(val(:,1),val(:,2)),disp(sys),port_label('input',1,'Address'),port_label('output',1,'Result'),port_label('output',2,'Error')
  Result : Outport
  Error : Outport  Port=2
  wires:
  S-Function Builder77/2 -> Error/1
  S-Function Builder77/1 -> Result/1
  Address/1 -> S-Function Builder77/1

== system ALL_SET_GET_SETUP_Funcitons_Library_2020a/Get_Functions/GetMotorDirection ==
  Address : Inport
  S-Function Builder82 : S-Function  Priority=3  FunctionName=GetMotorDirection  SFunctionModules=GetMotorDirection_wrapper  SFunctionDeploymentMode=off  EnableBusSupport=off  mask(S-Function Builder){}
      mask help: Simulink:masks:SFunctionBuilder_MD
      mask init: same as ALL_SET_GET_SETUP_Funcitons_Library_2020a/Get_Functions/Get3PhaseMotorAngle/S-Function Builder87
      settings: CopyFcn=set_param(gcbh,'LinkStatus','none')  OpenFcn=sfunctionwizard(gcbh)
      mask Display:
      | plot(val(:,1),val(:,2))
      | disp(sys)
      | port_label('input',1,'Address')
      | port_label('output',1,'Result')
      | port_label('output',2,'Error')
  Result : Outport
  Error : Outport  Port=2
  wires:
  S-Function Builder82/2 -> Error/1
  S-Function Builder82/1 -> Result/1
  Address/1 -> S-Function Builder82/1

== system ALL_SET_GET_SETUP_Funcitons_Library_2020a/Get_Functions/GetMotorInductance ==
  Address : Inport
  S-Function Builder65 : S-Function  Priority=3  FunctionName=GetMotorInductance  SFunctionModules=GetMotorInductance_wrapper  SFunctionDeploymentMode=off  EnableBusSupport=off  mask(S-Function Builder){}
      mask help: Simulink:masks:SFunctionBuilder_MD
      mask init: same as ALL_SET_GET_SETUP_Funcitons_Library_2020a/Get_Functions/Get3PhaseMotorAngle/S-Function Builder87
      settings: CopyFcn=set_param(gcbh,'LinkStatus','none')  OpenFcn=sfunctionwizard(gcbh)
      mask Display: plot(val(:,1),val(:,2)),disp(sys),port_label('input',1,'Address'),port_label('output',1,'Result'),port_label('output',2,'Error')
  Result : Outport
  Error : Outport  Port=2
  wires:
  S-Function Builder65/1 -> Result/1
  S-Function Builder65/2 -> Error/1
  Address/1 -> S-Function Builder65/1

== system ALL_SET_GET_SETUP_Funcitons_Library_2020a/Get_Functions/GetMotorPoleCounts ==
  Address : Inport
  S-Function Builder59 : S-Function  Priority=3  FunctionName=GetMotorPolesCounts  SFunctionModules=GetMotorPolesCounts_wrapper  SFunctionDeploymentMode=off  EnableBusSupport=off  mask(S-Function Builder){}
      mask help: Simulink:masks:SFunctionBuilder_MD
      mask init: same as ALL_SET_GET_SETUP_Funcitons_Library_2020a/Get_Functions/Get3PhaseMotorAngle/S-Function Builder87
      settings: CopyFcn=set_param(gcbh,'LinkStatus','none')  OpenFcn=sfunctionwizard(gcbh)
      mask Display:
      | plot(val(:,1),val(:,2))
      | disp(sys)
      | port_label('input',1,'Address')
      | port_label('output',1,'Result')
      | port_label('output',2,'Error')
  Result : Outport
  Error : Outport  Port=2
  wires:
  Address/1 -> S-Function Builder59/1
  S-Function Builder59/1 -> Result/1
  S-Function Builder59/2 -> Error/1

== system ALL_SET_GET_SETUP_Funcitons_Library_2020a/Get_Functions/GetMotorResistance ==
  Address : Inport
  S-Function Builder64 : S-Function  Priority=3  FunctionName=GetMotorResistance  SFunctionModules=GetMotorResistance_wrapper  SFunctionDeploymentMode=off  EnableBusSupport=off  mask(S-Function Builder){}
      mask help: Simulink:masks:SFunctionBuilder_MD
      mask init: same as ALL_SET_GET_SETUP_Funcitons_Library_2020a/Get_Functions/Get3PhaseMotorAngle/S-Function Builder87
      settings: CopyFcn=set_param(gcbh,'LinkStatus','none')  OpenFcn=sfunctionwizard(gcbh)
      mask Display: plot(val(:,1),val(:,2)),disp(sys),port_label('input',1,'Address'),port_label('output',1,'Result'),port_label('output',2,'Error')
  Result : Outport
  Error : Outport  Port=2
  wires:
  S-Function Builder64/1 -> Result/1
  Address/1 -> S-Function Builder64/1
  S-Function Builder64/2 -> Error/1

== system ALL_SET_GET_SETUP_Funcitons_Library_2020a/Get_Functions/GetMotorType ==
  Address : Inport
  S-Function Builder67 : S-Function  Priority=3  FunctionName=GetMotorType  SFunctionModules=GetMotorType_wrapper  SFunctionDeploymentMode=off  EnableBusSupport=off  mask(S-Function Builder){}
      mask help: Simulink:masks:SFunctionBuilder_MD
      mask init: same as ALL_SET_GET_SETUP_Funcitons_Library_2020a/Get_Functions/Get3PhaseMotorAngle/S-Function Builder87
      settings: CopyFcn=set_param(gcbh,'LinkStatus','none')  OpenFcn=sfunctionwizard(gcbh)
      mask Display:
      | plot(val(:,1),val(:,2))
      | disp(sys)
      | port_label('input',1,'Address')
      | port_label('output',1,'Result')
      | port_label('output',2,'Error')
  Result : Outport
  Error : Outport  Port=2
  wires:
  S-Function Builder67/1 -> Result/1
  S-Function Builder67/2 -> Error/1
  Address/1 -> S-Function Builder67/1

== system ALL_SET_GET_SETUP_Funcitons_Library_2020a/Get_Functions/GetObserverGainBldcPmsm ==
  Address : Inport
  S-Function Builder81 : S-Function  Priority=3  FunctionName=GetObserverGainBldcPmsm  SFunctionModules=GetObserverGainBldcPmsm_wrapper  SFunctionDeploymentMode=off  EnableBusSupport=off  mask(S-Function Builder){}
      mask help: Simulink:masks:SFunctionBuilder_MD
      mask init: same as ALL_SET_GET_SETUP_Funcitons_Library_2020a/Get_Functions/Get3PhaseMotorAngle/S-Function Builder87
      settings: CopyFcn=set_param(gcbh,'LinkStatus','none')  OpenFcn=sfunctionwizard(gcbh)
      mask Display: plot(val(:,1),val(:,2)),disp(sys),port_label('input',1,'Address'),port_label('output',1,'Result'),port_label('output',2,'Error')
  Result : Outport
  Error : Outport  Port=2
  wires:
  Address/1 -> S-Function Builder81/1
  S-Function Builder81/1 -> Result/1
  S-Function Builder81/2 -> Error/1

== system ALL_SET_GET_SETUP_Funcitons_Library_2020a/Get_Functions/GetObserverGainBldcPmsmUltrafast ==
  Address : Inport
  S-Function Builder83 : S-Function  Priority=3  FunctionName=GetObserverGainBldcPmsmUltrafast  SFunctionModules=GetObserverGainBldcPmsmUltrafast_wrapper  SFunctionDeploymentMode=off  EnableBusSupport=off  mask(S-Function Builder){}
      mask help: Simulink:masks:SFunctionBuilder_MD
      mask init: same as ALL_SET_GET_SETUP_Funcitons_Library_2020a/Get_Functions/Get3PhaseMotorAngle/S-Function Builder87
      settings: CopyFcn=set_param(gcbh,'LinkStatus','none')  OpenFcn=sfunctionwizard(gcbh)
      mask Display: plot(val(:,1),val(:,2)),disp(sys),port_label('input',1,'Address'),port_label('output',1,'Result'),port_label('output',2,'Error')
  Result : Outport
  Error : Outport  Port=2
  wires:
  S-Function Builder83/2 -> Error/1
  S-Function Builder83/1 -> Result/1
  Address/1 -> S-Function Builder83/1

== system ALL_SET_GET_SETUP_Funcitons_Library_2020a/Get_Functions/GetObserverGainDc ==
  Address : Inport
  S-Function Builder84 : S-Function  Priority=3  FunctionName=GetObserverGainDc  SFunctionModules=GetObserverGainDc_wrapper  SFunctionDeploymentMode=off  EnableBusSupport=off  mask(S-Function Builder){}
      mask help: Simulink:masks:SFunctionBuilder_MD
      mask init: same as ALL_SET_GET_SETUP_Funcitons_Library_2020a/Get_Functions/Get3PhaseMotorAngle/S-Function Builder87
      settings: CopyFcn=set_param(gcbh,'LinkStatus','none')  OpenFcn=sfunctionwizard(gcbh)
      mask Display: plot(val(:,1),val(:,2)),disp(sys),port_label('input',1,'Address'),port_label('output',1,'Result'),port_label('output',2,'Error')
  Result : Outport
  Error : Outport  Port=2
  wires:
  S-Function Builder84/2 -> Error/1
  S-Function Builder84/1 -> Result/1
  Address/1 -> S-Function Builder84/1
